simulink model "PV_Geno_VSC_GFL_634"  (R2024b)
settings: Solver=ode5  StartTime=0.0  StopTime=5  MaxStep=1e-4  RelTol=1e-6  AbsTol=1e-8
values from neighbouring files (symbols this model uses):
  a = 1.3    [init_para_with_symmtrc_loads.m]
  amp_ptb = amp_rel*Vp    [a01_scan_VSC_13_feeder.m]
  Cdc = 278e-3    (= 0.278)    [init_para_with_symmtrc_loads.m]
  fg = 60    [a01_scan_VSC_13_feeder.m]    (also in init_para_with_symmtrc_loads.m)
  Gn = 1000    [init_para_with_symmtrc_loads.m]
  Ipv_n = Isc_n*(Rp+Rs)/Rp    (= 8.21426513558)    [init_para_with_symmtrc_loads.m]
  Isc_n = 8.21    [init_para_with_symmtrc_loads.m]
  k = 1.3806503e-23    [init_para_with_symmtrc_loads.m]    (also in ypm_plot_compare_ana_meas.m = 2)
  KI = 0.0032    [init_para_with_symmtrc_loads.m]
  Ki_C = Rc/tau_C    (= 0.768)    [init_para_with_symmtrc_loads.m]
  Ki_DC = omega_DC^2*Cdc    [init_para_with_symmtrc_loads.m]
  Ki_P = 1/(Ki_pq*tau_P)    [init_para_with_symmtrc_loads.m]
  Ki_PLL = Kp_PLL/tau_PLL    [init_para_with_symmtrc_loads.m]
  Kp_C = Lc/tau_C    (= 0.020372)    [init_para_with_symmtrc_loads.m]
  Kp_DC = 2*xi_DC*omega_DC*Cdc    [init_para_with_symmtrc_loads.m]
  Kp_P = tau_C/(Ki_pq*tau_P)    [init_para_with_symmtrc_loads.m]
  Kp_PLL = xi_PLL*2*omega_PLL/Vp    [init_para_with_symmtrc_loads.m]
  KV = -0.123    [init_para_with_symmtrc_loads.m]
  KVmp = Vmp_n/Voc_n    (= 0.799392097264)    [init_para_with_symmtrc_loads.m]
  Lc = 20.372e-6    (= 2.0372e-05)    [init_para_with_symmtrc_loads.m]
  Np = 345    [init_para_with_symmtrc_loads.m]
  Ns = 45    [init_para_with_symmtrc_loads.m]
  Ns_cell = 54    [init_para_with_symmtrc_loads.m]
  phi_ptb = phi_ptb_vec(run)    [a01_scan_VSC_13_feeder.m]
  phs0 = mod(-w_ptb*t_start, 2*pi)    [a01_scan_VSC_13_feeder.m]
  psi_0 = 0    [a01_scan_VSC_13_feeder.m]
  q = 1.6021764e-19    [init_para_with_symmtrc_loads.m]
  Rc = 0.768e-3    (= 0.000768)    [init_para_with_symmtrc_loads.m]
  Rp = 425.405    [init_para_with_symmtrc_loads.m]
  Rs = 0.221    [init_para_with_symmtrc_loads.m]
  S_base_all = 1    [init_para_with_symmtrc_loads.m]
  t_start = t_settle    (= 0.5)    [a01_scan_VSC_13_feeder.m]
  Tn = 25    [init_para_with_symmtrc_loads.m]
  Ts = T_ctrl/n_ctrl    [a01_scan_VSC_13_feeder.m]    (also in init_para_with_symmtrc_loads.m = 5e-05)
  Vdc = 1200    [init_para_with_symmtrc_loads.m]
  Voc_n = 32.9    [init_para_with_symmtrc_loads.m]
  Vp = sqrt(2)*480/sqrt(3)    [a01_scan_VSC_13_feeder.m]    (also in init_para_with_symmtrc_loads.m = Ug*sqrt(2)/sqrt(3))
  w_ptb = 2*pi*fp    [a01_scan_VSC_13_feeder.m]
undefined symbols (not defined in the file or in its folder): Amp_ptb_A, Amp_ptb_B, Amp_ptb_C, DiscIntNeverNeededParam, frq_ptb_A, frq_ptb_B, frq_ptb_C, j, para_PVgeno, phs_ptb_A, phs_ptb_B, phs_ptb_C
libraries: spsControlledVoltageSourceLib x6, slpidlib x5, spsSeriesRLCBranchLib x4, spsPower3phInstantaneousLib x2, spsabctoAlphaBetaZeroLib x2, spsCurrentMeasurementLib x2, spsControlledCurrentSourceLib x2, spsGroundLib x1, spsVoltageMeasurementLib x1, spsThreePhaseVIMeasurementLib x1, spsThreePhaseParallelRLCLoadLib x1, spsThreePhaseSourceLib x1
(part 2 of 2)

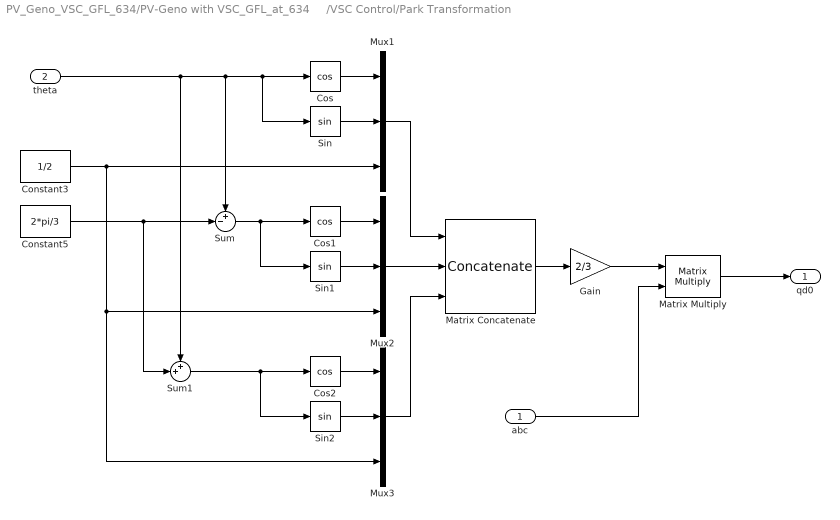
== system PV_Geno_VSC_GFL_634/PV-Geno with VSC_GFL_at_634     /VSC Control/Park Transformation ==
  abc : Inport
  theta : Inport  Port=2
  Constant3 : Constant  Value=1/2
  Constant5 : Constant  Value=2*pi/3
  Cos : Trigonometry  Operator=cos
  Cos1 : Trigonometry  Operator=cos
  Cos2 : Trigonometry  Operator=cos
  Gain : Gain  Gain=2/3
  Matrix Concatenate : Concatenate  NumInputs=3  Mode=Multidimensional array  ConcatenateDimension=2
  Matrix Multiply : Product  Multiplication=Matrix(*)
  Mux1 : Mux  Inputs=3
  Mux2 : Mux  Inputs=3
  Mux3 : Mux  Inputs=3
  Sin : Trigonometry
  Sin1 : Trigonometry
  Sin2 : Trigonometry
  Sum : Sum  Inputs=+-|
  Sum1 : Sum  Inputs=++|
  qd0 : Outport
  wires:
  Sum1/1 -> Sin2/1, Cos2/1
  abc/1 -> Matrix Multiply/2
  Cos/1 -> Mux1/1
  Gain/1 -> Matrix Multiply/1
  theta/1 -> Sum1/1, Sum/1, Cos/1, Sin/1
  Constant3/1 -> Mux3/3, Mux2/3, Mux1/3
  Sin2/1 -> Mux3/2
  Sin/1 -> Mux1/2
  Mux2/1 -> Matrix Concatenate/2
  Sum/1 -> Sin1/1, Cos1/1
  Cos2/1 -> Mux3/1
  Mux1/1 -> Matrix Concatenate/1
  Cos1/1 -> Mux2/1
  Mux3/1 -> Matrix Concatenate/3
  Sin1/1 -> Mux2/2
  Matrix Concatenate/1 -> Gain/1
  Matrix Multiply/1 -> qd0/1
  Constant5/1 -> Sum/2, Sum1/2

== system PV_Geno_VSC_GFL_634/PV-Geno with VSC_GFL_at_634     /VSC Control/Q Control ==
  Q_ref : Inport
  v_abc : Inport  Port=2
  i_abc : Inport  Port=3
  Mux1 : Mux  Inputs=2
  PID Controller3 : slpidlib/PID Controller  Controller=PI  Form=Parallel  TimeDomain=Discrete-time  UseExternalTs=off  SampleTime=Ts  IntegratorMethod=Forward Euler  FilterMethod=Forward Euler  ControllerParametersSource=internal  P=Kp_P  I=Ki_P  UseKiTs=off  D=0  UseExternalDerivativeSource=off  N=100  UseFilter=on  TunerSelectOption=Transfer Function Based (PID Tuner App)  InitialConditionSource=internal  InitialConditionForIntegrator=0  InitialConditionForFilter=0  DifferentiatorICPrevScaledInput=0  ExternalReset=none  TrackingMode=off  Kt=1  LimitOutput=off  SatLimitsSource=internal  UpperSaturationLimit=inf  LowerSaturationLimit=-inf  LinearizeAsGain=on  AntiWindupMode=none  Kb=1  LimitIntegrator=off  UpperIntegratorSaturationLimit=inf  LowerIntegratorSaturationLimit=-inf  POutMin=[]  POutMax=[]  IOutMin=[]  IOutMax=[]  DOutMin=[]  DOutMax=[]  NOutMin=[]  NOutMax=[]  SumOutMin=[]  SumOutMax=[]  SaturationOutMin=[]  SaturationOutMax=[]  PParamMin=[]  PParamMax=[]  IParamMin=[]  IParamMax=[]  DParamMin=[]  DParamMax=[]  NParamMin=[]  NParamMax=[]  KbParamMin=[]  KbParamMax=[]  KtParamMin=[]  KtParamMax=[]  KbOutMin=[]  KbOutMax=[]  KtOutMin=[]  KtOutMax=[]  IntegratorOutMin=[]  IntegratorOutMax=[]  FilterOutMin=[]  FilterOutMax=[]  SumI1OutMin=[]  SumI1OutMax=[]  SumI2OutMin=[]  SumI2OutMax=[]  SumI3OutMin=[]  SumI3OutMax=[]  SumI4OutMin=[]  SumI4OutMax=[]  SumDOutMin=[]  SumDOutMax=[]  DifferentiatorOutMin=[]  DifferentiatorOutMax=[]  FilterDiffOutCoefMin=[]  FilterDiffOutCoefMax=[]  ReciprocalOutMin=[]  ReciprocalOutMax=[]  SumDenOutMin=[]  SumDenOutMax=[]  SumNumOutMin=[]  SumNumOutMax=[]  DivideOutMin=[]  DivideOutMax=[]  UdiffTsProdOutMin=[]  UdiffTsProdOutMax=[]  NTsProdOutMin=[]  NTsProdOutMax=[]  UintegralTsProdOutMin=[]  UintegralTsProdOutMax=[]  UngainTsProdOutMin=[]  UngainTsProdOutMax=[]  ClampingZeroOutDataTypeStr=Inherit: Inherit via back propagation  ClampingZeroOutMin=[]  ClampingZeroOutMax=[]  FilterDenConstantOutDataTypeStr=Inherit: Inherit via back propagation  FilterDenConstantOutMin=[]  FilterDenConstantOutMax=[]  PCopyOutDataTypeStr=Inherit: Inherit via back propagation  PCopyOutMin=[]  PCopyOutMax=[]  NCopyOutDataTypeStr=Inherit: Inherit via back propagation  NCopyOutMin=[]  NCopyOutMax=[]  IntegratorContinuousStateAttributes=''  IntegratorStateMustResolveToSignalObject=off  IntegratorRTWStateStorageClass=Auto  FilterContinuousStateAttributes=''  FilterStateMustResolveToSignalObject=off  FilterRTWStateStorageClass=Auto  ParallelPVariant=InternalParameters  IdealPVariant=Disabled  IVariant=InternalParameters  DVariant=Disabled  IntegratorVariant=Discrete  SatVariant=Disabled  AWVariant=Passthrough  PCopyVariant=Disabled  TRVariant=Disabled  FdbkBlocksVariant=Forward  IdealPFdbkVariant=Disabled  SatFdbkVariant=Disabled  DerivativeFilterVariant=Disabled  NVariant=Disabled  NCopyVariant=Disabled_SignalSpec  FilterICVariant=Disabled  IntegratorICVariant=InternalICs  ExternalResetVariant=Disabled  TRSumVariant=Passthrough  SumFdbkVariant=Disabled  SumVariant=Sum_PI  TsampFilterVariant=InternalTs  TsampNgainVariant=Passthrough  TsampIntegralVariant=Disabled_SignalSpec  ExternalSaturationOutDataTypeStr=Inherit: Same as second input  DerivativeSourceVariant=Disabled  PreIntVariant=InternalPreInt
  "Power (3ph, Instantaneous)" : spsPower3phInstantaneousLib/Power (3ph, Instantaneous)
  Sum3 : Sum  Inputs=|+-
  id_ref : Outport
  PQ : Outport  Port=2
  tag scope: y_PI_QC=global
  wires:
  Q_ref/1 -> Sum3/1
  "Power (3ph, Instantaneous)"/1 -> Mux1/1
  Sum3/1 -> PID Controller3/1
  i_abc/1 -> "Power (3ph, Instantaneous)"/2
  v_abc/1 -> "Power (3ph, Instantaneous)"/1
  "Power (3ph, Instantaneous)"/2 -> Sum3/2, Mux1/2
  Mux1/1 -> PQ/1
  PID Controller3/1 -> [y_PI_QC], id_ref/1

== system PV_Geno_VSC_GFL_634/PV-Geno with VSC_GFL_at_634     /VSC Control/Current Control/Inverse Park Transformation ==
  qd0 : Inport
  theta : Inport  Port=2
  Constant2 : Constant
  Constant3 : Constant  Value=2*pi/3
  Cos : Trigonometry  Operator=cos
  Matrix Concatenate : Concatenate  NumInputs=3  Mode=Multidimensional array  ConcatenateDimension=2
  Matrix Multiply : Product  Multiplication=Matrix(*)
  Mux1 : Mux  Inputs=3
  Mux2 : Mux  Inputs=3
  Sin : Trigonometry
  Sum : Sum  Inputs=+-|
  Sum1 : Sum  Inputs=++|
  abc : Outport
  wires:
  Constant3/1 -> Sum/2, Sum1/2
  theta/1 -> Mux1/1, Sum1/1, Sum/1
  qd0/1 -> Matrix Multiply/2
  Sum/1 -> Mux1/2
  Sum1/1 -> Mux1/3
  Matrix Multiply/1 -> abc/1
  Mux2/1 -> Matrix Concatenate/3
  Matrix Concatenate/1 -> Matrix Multiply/1
  Mux1/1 -> Cos/1, Sin/1
  Cos/1 -> Matrix Concatenate/1
  Constant2/1 -> Mux2/2, Mux2/3, Mux2/1
  Sin/1 -> Matrix Concatenate/2

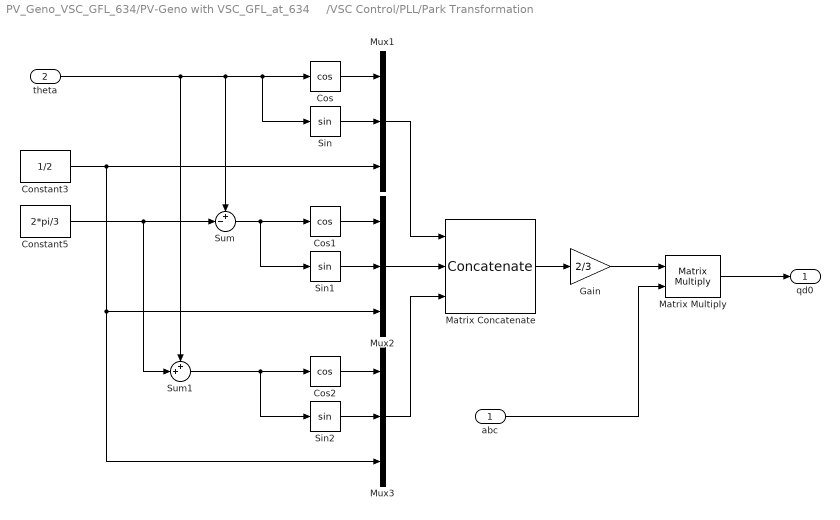
== system PV_Geno_VSC_GFL_634/PV-Geno with VSC_GFL_at_634     /VSC Control/PLL/Park Transformation ==
  abc : Inport
  theta : Inport  Port=2
  Constant3 : Constant  Value=1/2
  Constant5 : Constant  Value=2*pi/3
  Cos : Trigonometry  Operator=cos
  Cos1 : Trigonometry  Operator=cos
  Cos2 : Trigonometry  Operator=cos
  Gain : Gain  Gain=2/3
  Matrix Concatenate : Concatenate  NumInputs=3  Mode=Multidimensional array  ConcatenateDimension=2
  Matrix Multiply : Product  Multiplication=Matrix(*)
  Mux1 : Mux  Inputs=3
  Mux2 : Mux  Inputs=3
  Mux3 : Mux  Inputs=3
  Sin : Trigonometry
  Sin1 : Trigonometry
  Sin2 : Trigonometry
  Sum : Sum  Inputs=+-|
  Sum1 : Sum  Inputs=++|
  qd0 : Outport
  wires:
  Constant5/1 -> Sum1/2, Sum/2
  Matrix Multiply/1 -> qd0/1
  Matrix Concatenate/1 -> Gain/1
  Sin1/1 -> Mux2/2
  Mux3/1 -> Matrix Concatenate/3
  Cos1/1 -> Mux2/1
  Mux1/1 -> Matrix Concatenate/1
  Cos2/1 -> Mux3/1
  Sum/1 -> Cos1/1, Sin1/1
  Mux2/1 -> Matrix Concatenate/2
  Sin/1 -> Mux1/2
  Sin2/1 -> Mux3/2
  Constant3/1 -> Mux1/3, Mux2/3, Mux3/3
  theta/1 -> Sin/1, Cos/1, Sum/1, Sum1/1
  Gain/1 -> Matrix Multiply/1
  Cos/1 -> Mux1/1
  abc/1 -> Matrix Multiply/2
  Sum1/1 -> Cos2/1, Sin2/1
